simulink model "HILClimbers_LED_Rear_Light_Module_V5"  (R2021a)
settings: Solver=VariableStepAuto  StartTime=0.0  StopTime=inf  RelTol=1e-3
model workspace (MAT data in the model file):
  brake = 0
settings Model: Creator=Sai229  LastModifiedBy=Sai229

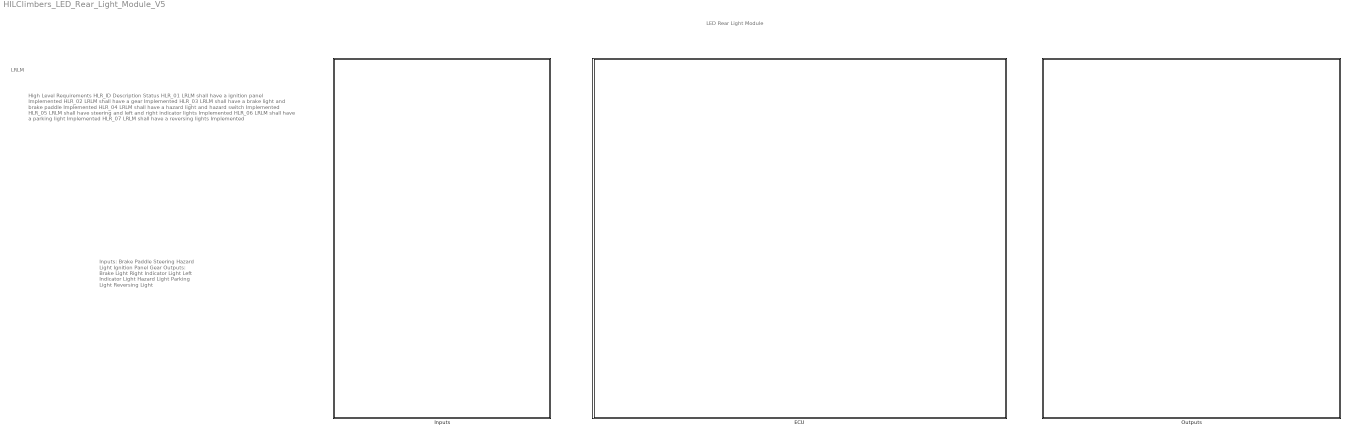
== system HILClimbers_LED_Rear_Light_Module_V5 ==
  note: LRLM
  note: Inputs:
      | Brake Paddle
      | Steering
      | Hazard Light
      | Ignition Panel
      | Gear
      |
      | Outputs:
      | Brake Light
      | Right Indicator Light
      | Left Indicator Light
      | Hazard Light
      | Parking Light
      | Reversing Light
  note: High Level Requirements
      |
      | HLR_ID
      | Description
      | Status
      |
      | HLR_01
      | LRLM shall have a ignition panel
      | Implemented
      |
      | HLR_02
      | LRLM shall have a gear
      | Implemented
      |
      | HLR_03
      | LRLM shall have a brake light and brake paddle
      | Implemented
      |
      | HLR_04
      | LRLM shall have a hazard light and hazard switch
      | Implemented
      |
      | HLR_05
      | LRLM shall have steering and left and right indicator lights
      | Implemented
      |
      | HLR_06
      | LRLM shall have a parking light
      | Implemented
      |
      | HLR_07
      | LRLM shall have a reversing lights
      | Implemented
  note: LED Rear Light Module
  ECU : Subsystem  ReferencedSubsystem=LRLM_ECU  time_period=1
  Inputs : Subsystem
  Outputs : Subsystem

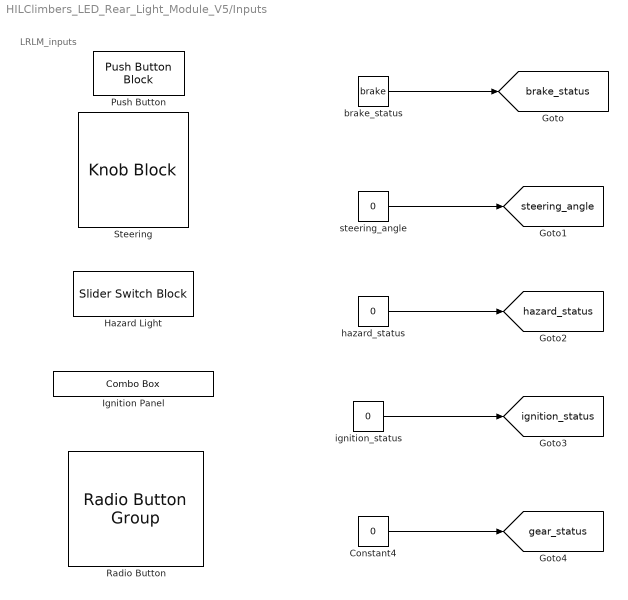
== system HILClimbers_LED_Rear_Light_Module_V5/Inputs ==
  note: LRLM_inputs
  Constant4 : Constant  Value=0
  Hazard Light : SliderSwitchBlock  LabelPosition=Hide
      settings: Values={{'Off', 'On'}, [0 1]}
  Ignition Panel : ComboBox  LabelPosition=Hide  SelectedLabel=Key Not Inserted
      settings: Values={{'Key Not Inserted', 'Key Inserted', 'Pre-Ignition', 'Vehicle Started'}, [0 1 2 3]}
  Push Button : PushButtonBlock  ButtonText=Brake
  Radio Button : RadioButtonGroup  LabelPosition=Hide  SelectedLabel=Neutral  ButtonGroupName=Gear
      settings: Values={{'Neutral', 'Drive', 'Park', 'Reverse'}, [0 1 2 3]}
  Steering : KnobBlock  LabelPosition=Hide  ScaleMin=-50  ScaleMax=50  TickInterval=10
  brake_status : Constant  Value=brake
  hazard_status : Constant  Value=0
  ignition_status : Constant  Value=0
  steering_angle : Constant  Value=0
  tag scope: brake_status=global, gear_status=global, hazard_status=global, ignition_status=global, steering_angle=global
  wires:
  hazard_status/1 -> [hazard_status]
  steering_angle/1 -> [steering_angle]
  brake_status/1 -> [brake_status]
  ignition_status/1 -> [ignition_status]
  Constant4/1 -> [gear_status]

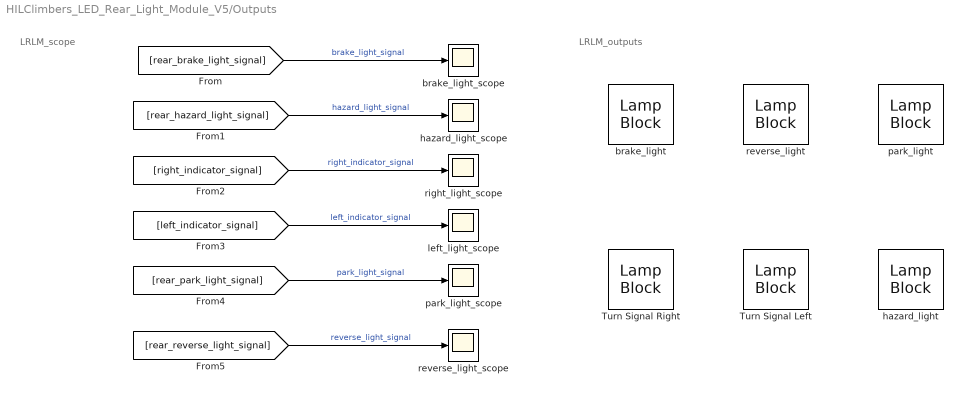
== system HILClimbers_LED_Rear_Light_Module_V5/Outputs ==
  note: LRLM_scope
  note: LRLM_outputs
  Turn Signal Left : LampBlock  LabelPosition=Hide  Icon=TurnSignalLeft
  Turn Signal Right : LampBlock  LabelPosition=Hide  Icon=TurnSignalRight
  brake_light : LampBlock  LabelPosition=Hide  Icon=LightingSwitch
  brake_light_scope : Scope
  hazard_light : LampBlock  LabelPosition=Hide  Icon=Hazards
  hazard_light_scope : Scope
  left_light_scope : Scope
  park_light : LampBlock  Icon=ParkingAssistance
  park_light_scope : Scope
  reverse_light : LampBlock  Icon=RearFogLight
  reverse_light_scope : Scope
  right_light_scope : Scope
  wires:
  [rear_brake_light_signal] -> brake_light_scope/1  "brake_light_signal"
  [rear_hazard_light_signal] -> hazard_light_scope/1  "hazard_light_signal"
  [rear_park_light_signal] -> park_light_scope/1  "park_light_signal"
  [rear_reverse_light_signal] -> reverse_light_scope/1  "reverse_light_signal"
  [right_indicator_signal] -> right_light_scope/1  "right_indicator_signal"
  [left_indicator_signal] -> left_light_scope/1  "left_indicator_signal"
